simulink model "test_tq_distbn_srv"  (R2019b)
settings: Solver=FixedStepAuto  StartTime=0.0  StopTime=100  FixedStep=0.001  RelTol=1e-3
libraries: simulink x1
settings Model: Creator=DIS3SI  LastModifiedBy=DIS3SI

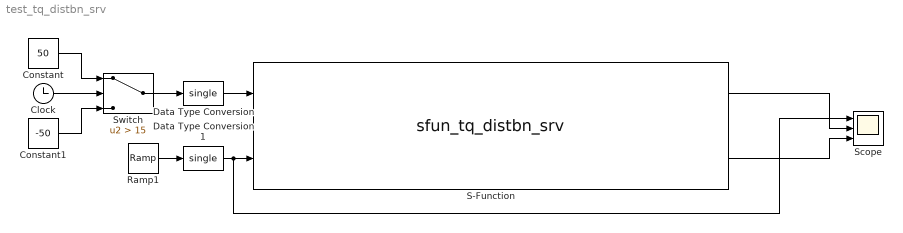
== system test_tq_distbn_srv ==
  Clock : Clock
  Constant : Constant  Value=50
  Constant1 : Constant  Value=-50
  Data Type Conversion : DataTypeConversion  OutDataTypeStr=single
  Data Type Conversion1 : DataTypeConversion  OutDataTypeStr=single
  Ramp1 : simulink/Sources/Ramp  slope=10  start=0  InitialOutput=-200
  S-Function : S-Function  FunctionName=sfun_tq_distbn_srv  SFunctionDeploymentMode=off  EnableBusSupport=off
      mask Display:
      | disp('tq_distbn_srv');
      | port_label('input', 1, 'powertrain_tq_recuperation_capacity_actual_Nm');
      | port_label('input', 2, 'powertrain_tq_tar_total_Nm');
      | 
      | port_label('output', 1, 'tq_distbn_srv_tq_tar_pt_Nm');
      | port_label('output', 2, 'out_tq_distbn_srv_tq_tar_brk_Nm');
  Scope : Scope  NumInputPorts=3
  Switch : Switch  Criteria=u2 > Threshold  Threshold=15
  wires:
  Switch/1 -> Data Type Conversion/1
  Ramp1/1 -> Data Type Conversion1/1
  S-Function/1 -> Scope/2
  S-Function/2 -> Scope/3
  Data Type Conversion/1 -> S-Function/1
  Data Type Conversion1/1 -> Scope/1, S-Function/2
  Constant/1 -> Switch/1
  Constant1/1 -> Switch/3
  Clock/1 -> Switch/2
